simulink library "cdsSqrt"  (Simulink 7.8)
settings: Solver=ode45  SolverMode=SingleTasking  StartTime=0.0  StopTime=10.0  RelTol=1e-3
settings Model: Creator=rolf  LastModifiedBy=rolf

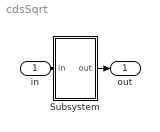
== system cdsSqrt ==
  in : Inport
  Subsystem : Subsystem
  out : Outport
  wires:
  Subsystem/1(out) -> out/1
  in/1 -> Subsystem/1(in)

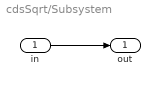
== system cdsSqrt/Subsystem ==
  in : Inport
  out : Outport
  wires:
  in/1 -> out/1
